simulink model "Hell_ix_Functional_Architecture"  (R2022b)
settings: Solver=VariableStepAuto  StartTime=0.0  StopTime=10.0  RelTol=1e-3
settings Model: Creator=Daniel Sotelo  LastModifiedBy=Daniel Sotelo

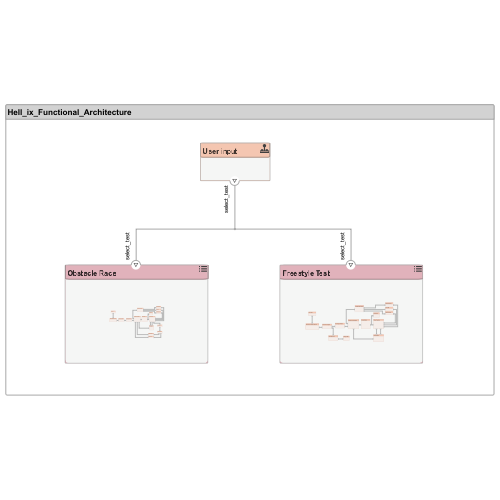
[thumbnail: Simulink's stored preview of the top-level diagram]
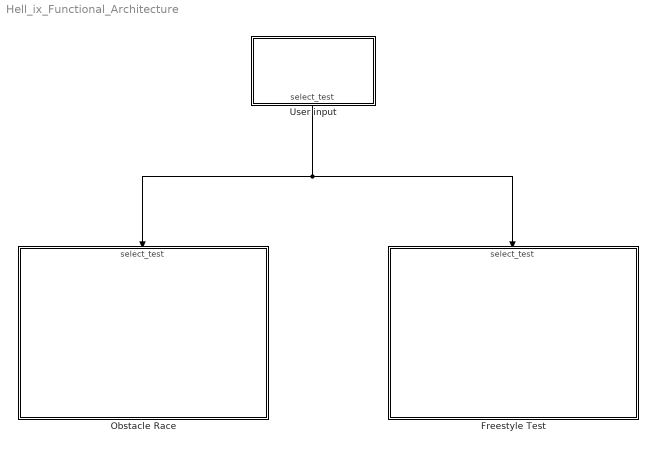
== system Hell_ix_Functional_Architecture ==
  Freestyle Test : Subsystem
      settings: PortSchema="{\"entries\":[{\"content\":{\"headerSize\":26,\"margin\":15,\"minimumSpacing\":25,\"sides\":[{\"content\":{\"connectorIds\":[]},\"type\":\"ConnectorPlacement.EquallySpacedRectSide\",\"uuid\":\"e97e1fd1-9f1b-43cc-bf15-a23fe97b9f57\"},{\"content\":{\"connectorIds\":[],\"side\":\"RIGHT\"},\"type\":\"ConnectorPlacement.EquallySpacedRectSide\",\"uuid\":\"b384b9c5-fcee-4054-b020-18cc4d409726\"},{\"content\":{\"connectorIds\":[\"In1\"],\"side\":\"TOP\"},\"type\":\"ConnectorPlacement.EquallySpacedRectSide\",\"uuid\":\"0ff74274-cc13-4bc9-ab97-befa0144ddb0\"}]},\"type\":\"ConnectorPlacement.EquallySpacedConnector\",\"uuid\":\"32a64cae-dc0e-47e5-be72-f6041fa7e3a1\"}],\"packageUris\":[\"http://schema.mathworks.com/mf0/Connector/R2020b\"],\"version\":\"1.0\"}"
  Obstacle Race : Subsystem
      settings: PortSchema="{\"entries\":[{\"content\":{\"headerSize\":26,\"margin\":15,\"minimumSpacing\":25,\"sides\":[{\"content\":{\"connectorIds\":[]},\"type\":\"ConnectorPlacement.EquallySpacedRectSide\",\"uuid\":\"e97e1fd1-9f1b-43cc-bf15-a23fe97b9f57\"},{\"content\":{\"connectorIds\":[],\"side\":\"RIGHT\"},\"type\":\"ConnectorPlacement.EquallySpacedRectSide\",\"uuid\":\"b384b9c5-fcee-4054-b020-18cc4d409726\"},{\"content\":{\"connectorIds\":[\"In1\"],\"side\":\"TOP\"},\"type\":\"ConnectorPlacement.EquallySpacedRectSide\",\"uuid\":\"0ff74274-cc13-4bc9-ab97-befa0144ddb0\"}]},\"type\":\"ConnectorPlacement.EquallySpacedConnector\",\"uuid\":\"32a64cae-dc0e-47e5-be72-f6041fa7e3a1\"}],\"packageUris\":[\"http://schema.mathworks.com/mf0/Connector/R2020b\"],\"version\":\"1.0\"}"
  User input : Subsystem
      settings: PortSchema="{\"entries\":[{\"content\":{\"headerSize\":26,\"margin\":15,\"minimumSpacing\":25,\"sides\":[{\"content\":{\"connectorIds\":[]},\"type\":\"ConnectorPlacement.EquallySpacedRectSide\",\"uuid\":\"30ce29f3-0e24-4ebf-9153-3e6ba72d02a3\"},{\"content\":{\"connectorIds\":[],\"side\":\"RIGHT\"},\"type\":\"ConnectorPlacement.EquallySpacedRectSide\",\"uuid\":\"fe9b11ce-d1c5-4b81-91f9-8a01d2df3f9c\"},{\"content\":{\"connectorIds\":[],\"side\":\"TOP\"},\"type\":\"ConnectorPlacement.EquallySpacedRectSide\",\"uuid\":\"b1de80d7-4ec1-40a0-acfa-b891e3e0d07e\"},{\"content\":{\"connectorIds\":[\"Out1\"],\"side\":\"BOTTOM\"},\"type\":\"ConnectorPlacement.EquallySpacedRectSide\",\"uuid\":\"e3e43ed0-9352-4cb6-b8e2-474aa3905c46\"}]},\"type\":\"ConnectorPlacement.EquallySpacedConnector\",\"uuid\":\"2db1e156-8200-4f9d-beaf-fd6631afb9bb\"}],\"packageUris\":[\"http://schema.mathworks.com/mf0/Connector/R2020b\"],\"version\":\"1.0\"}"
  wires:
  User input/1(select_test) -> Freestyle Test/1(select_test), Obstacle Race/1(select_test)

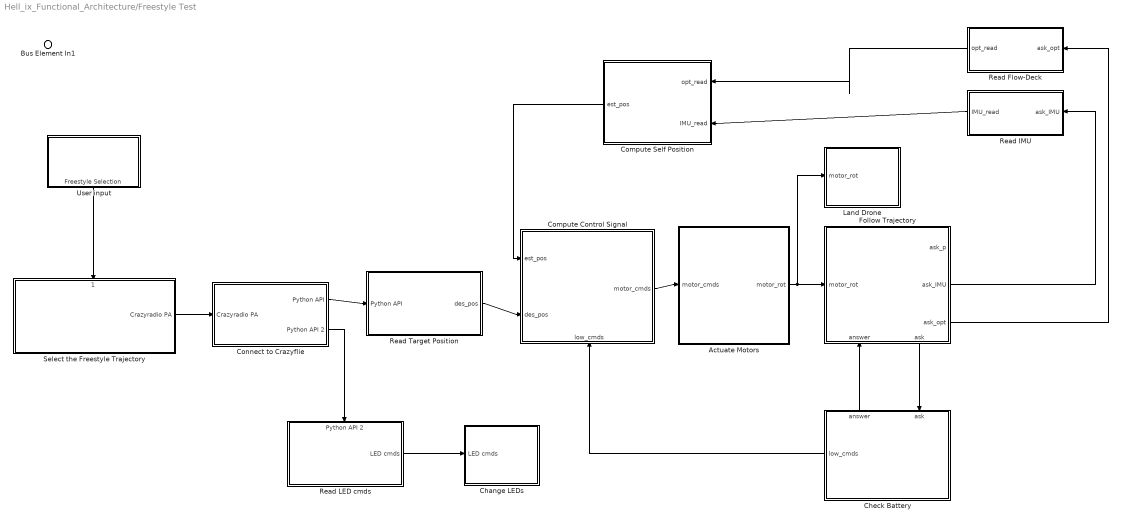
== system Hell_ix_Functional_Architecture/Freestyle Test ==
  Bus Element In1 : Inport  PortName=select_test
  Actuate Motors : Subsystem
      settings: PortSchema="{\"entries\":[{\"content\":{\"headerSize\":26,\"margin\":15,\"minimumSpacing\":25,\"sides\":[{\"content\":{\"connectorIds\":[\"In1\"]},\"type\":\"ConnectorPlacement.EquallySpacedRectSide\",\"uuid\":\"30ce29f3-0e24-4ebf-9153-3e6ba72d02a3\"},{\"content\":{\"connectorIds\":[\"Out1\"],\"side\":\"RIGHT\"},\"type\":\"ConnectorPlacement.EquallySpacedRectSide\",\"uuid\":\"fe9b11ce-d1c5-4b81-91f9-8a01d2df3f9c\"},{\"content\":{\"connectorIds\":[],\"side\":\"TOP\"},\"type\":\"ConnectorPlacement.EquallySpacedRectSide\",\"uuid\":\"b1de80d7-4ec1-40a0-acfa-b891e3e0d07e\"},{\"content\":{\"connectorIds\":[],\"side\":\"BOTTOM\"},\"type\":\"ConnectorPlacement.EquallySpacedRectSide\",\"uuid\":\"15269a5b-ba8a-48cb-be68-3964bc387354\"}]},\"type\":\"ConnectorPlacement.EquallySpacedConnector\",\"uuid\":\"2db1e156-8200-4f9d-beaf-fd6631afb9bb\"}],\"packageUris\":[\"http://schema.mathworks.com/mf0/Connector/R2020b\"],\"version\":\"1.0\"}"
  Change LEDs : Subsystem
      settings: PortSchema="{\"entries\":[{\"content\":{\"headerSize\":26,\"margin\":15,\"minimumSpacing\":25,\"sides\":[{\"content\":{\"connectorIds\":[\"In1\"]},\"type\":\"ConnectorPlacement.EquallySpacedRectSide\",\"uuid\":\"30ce29f3-0e24-4ebf-9153-3e6ba72d02a3\"},{\"content\":{\"connectorIds\":[],\"side\":\"RIGHT\"},\"type\":\"ConnectorPlacement.EquallySpacedRectSide\",\"uuid\":\"fe9b11ce-d1c5-4b81-91f9-8a01d2df3f9c\"},{\"content\":{\"connectorIds\":[],\"side\":\"TOP\"},\"type\":\"ConnectorPlacement.EquallySpacedRectSide\",\"uuid\":\"b1de80d7-4ec1-40a0-acfa-b891e3e0d07e\"}]},\"type\":\"ConnectorPlacement.EquallySpacedConnector\",\"uuid\":\"2db1e156-8200-4f9d-beaf-fd6631afb9bb\"}],\"packageUris\":[\"http://schema.mathworks.com/mf0/Connector/R2020b\"],\"version\":\"1.0\"}"
  Check Battery : Subsystem
      settings: PortSchema="{\"entries\":[{\"content\":{\"headerSize\":26,\"margin\":15,\"minimumSpacing\":25,\"sides\":[{\"content\":{\"connectorIds\":[\"Out1\"]},\"type\":\"ConnectorPlacement.EquallySpacedRectSide\",\"uuid\":\"30ce29f3-0e24-4ebf-9153-3e6ba72d02a3\"},{\"content\":{\"connectorIds\":[],\"side\":\"RIGHT\"},\"type\":\"ConnectorPlacement.EquallySpacedRectSide\",\"uuid\":\"fe9b11ce-d1c5-4b81-91f9-8a01d2df3f9c\"},{\"content\":{\"connectorIds\":[\"Out2\",\"In1\"],\"side\":\"TOP\"},\"type\":\"ConnectorPlacement.EquallySpacedRectSide\",\"uuid\":\"b1de80d7-4ec1-40a0-acfa-b891e3e0d07e\"}]},\"type\":\"ConnectorPlacement.EquallySpacedConnector\",\"uuid\":\"2db1e156-8200-4f9d-beaf-fd6631afb9bb\"}],\"packageUris\":[\"http://schema.mathworks.com/mf0/Connector/R2020b\"],\"version\":\"1.0\"}"
  Compute Control Signal : Subsystem
      settings: PortSchema="{\"entries\":[{\"content\":{\"headerSize\":26,\"margin\":15,\"minimumSpacing\":25,\"sides\":[{\"content\":{\"connectorIds\":[\"In2\",\"In3\"]},\"type\":\"ConnectorPlacement.EquallySpacedRectSide\",\"uuid\":\"30ce29f3-0e24-4ebf-9153-3e6ba72d02a3\"},{\"content\":{\"connectorIds\":[\"Out1\"],\"side\":\"RIGHT\"},\"type\":\"ConnectorPlacement.EquallySpacedRectSide\",\"uuid\":\"fe9b11ce-d1c5-4b81-91f9-8a01d2df3f9c\"},{\"content\":{\"connectorIds\":[],\"side\":\"TOP\"},\"type\":\"ConnectorPlacement.EquallySpacedRectSide\",\"uuid\":\"b1de80d7-4ec1-40a0-acfa-b891e3e0d07e\"},{\"content\":{\"connectorIds\":[\"In1\"],\"side\":\"BOTTOM\"},\"type\":\"ConnectorPlacement.EquallySpacedRectSide\",\"uuid\":\"15269a5b-ba8a-48cb-be68-3964bc387354\"}]},\"type\":\"ConnectorPlacement.EquallySpacedConnector\",\"uuid\":\"2db1e156-8200-4f9d-beaf-fd6631afb9bb\"}],\"packageUris\":[\"http://schema.mathworks.com/mf0/Connector/R2020b\"],\"version\":\"1.0\"}"
  Compute Self Position : Subsystem
      settings: PortSchema="{\"entries\":[{\"content\":{\"headerSize\":26,\"margin\":15,\"minimumSpacing\":25,\"sides\":[{\"content\":{\"connectorIds\":[\"Out1\"]},\"type\":\"ConnectorPlacement.EquallySpacedRectSide\",\"uuid\":\"30ce29f3-0e24-4ebf-9153-3e6ba72d02a3\"},{\"content\":{\"connectorIds\":[\"In1\",\"In2\"],\"side\":\"RIGHT\"},\"type\":\"ConnectorPlacement.EquallySpacedRectSide\",\"uuid\":\"fe9b11ce-d1c5-4b81-91f9-8a01d2df3f9c\"},{\"content\":{\"connectorIds\":[],\"side\":\"TOP\"},\"type\":\"ConnectorPlacement.EquallySpacedRectSide\",\"uuid\":\"b1de80d7-4ec1-40a0-acfa-b891e3e0d07e\"},{\"content\":{\"connectorIds\":[],\"side\":\"BOTTOM\"},\"type\":\"ConnectorPlacement.EquallySpacedRectSide\",\"uuid\":\"463c5264-2d4b-41d6-b420-fe60d6cb1965\"}]},\"type\":\"ConnectorPlacement.EquallySpacedConnector\",\"uuid\":\"2db1e156-8200-4f9d-beaf-fd6631afb9bb\"}],\"packageUris\":[\"http://schema.mathworks.com/mf0/Connector/R2020b\"],\"version\":\"1.0\"}"
  Connect to Crazyflie : Subsystem
      settings: PortSchema="{\"entries\":[{\"content\":{\"headerSize\":26,\"margin\":15,\"minimumSpacing\":25,\"sides\":[{\"content\":{\"connectorIds\":[\"In1\"]},\"type\":\"ConnectorPlacement.EquallySpacedRectSide\",\"uuid\":\"30ce29f3-0e24-4ebf-9153-3e6ba72d02a3\"},{\"content\":{\"connectorIds\":[\"Out1\",\"Out2\"],\"side\":\"RIGHT\"},\"type\":\"ConnectorPlacement.EquallySpacedRectSide\",\"uuid\":\"fe9b11ce-d1c5-4b81-91f9-8a01d2df3f9c\"},{\"content\":{\"connectorIds\":[],\"side\":\"TOP\"},\"type\":\"ConnectorPlacement.EquallySpacedRectSide\",\"uuid\":\"b1de80d7-4ec1-40a0-acfa-b891e3e0d07e\"}]},\"type\":\"ConnectorPlacement.EquallySpacedConnector\",\"uuid\":\"2db1e156-8200-4f9d-beaf-fd6631afb9bb\"}],\"packageUris\":[\"http://schema.mathworks.com/mf0/Connector/R2020b\"],\"version\":\"1.0\"}"
  Follow Trajectory : Subsystem
      settings: PortSchema="{\"entries\":[{\"content\":{\"headerSize\":26,\"margin\":15,\"minimumSpacing\":25,\"sides\":[{\"content\":{\"connectorIds\":[\"In2\"]},\"type\":\"ConnectorPlacement.EquallySpacedRectSide\",\"uuid\":\"30ce29f3-0e24-4ebf-9153-3e6ba72d02a3\"},{\"content\":{\"connectorIds\":[\"Out2\",\"Out1\",\"Out3\"],\"side\":\"RIGHT\"},\"type\":\"ConnectorPlacement.EquallySpacedRectSide\",\"uuid\":\"fe9b11ce-d1c5-4b81-91f9-8a01d2df3f9c\"},{\"content\":{\"connectorIds\":[],\"side\":\"TOP\"},\"type\":\"ConnectorPlacement.EquallySpacedRectSide\",\"uuid\":\"b1de80d7-4ec1-40a0-acfa-b891e3e0d07e\"},{\"content\":{\"connectorIds\":[\"In1\",\"Out4\"],\"side\":\"BOTTOM\"},\"type\":\"ConnectorPlacement.EquallySpacedRectSide\",\"uuid\":\"61505f5d-ae4a-4fe0-ac47-0fc326909193\"}]},\"type\":\"ConnectorPlacement.EquallySpacedConnector\",\"uuid\":\"2db1e156-8200-4f9d-beaf-fd6631afb9bb\"}],\"packageUris\":[\"http://schema.mathworks.com/mf0/Connector/R2020b\"],\"version\":\"1.0\"}"
  Land Drone : Subsystem
      settings: PortSchema="{\"entries\":[{\"content\":{\"headerSize\":26,\"margin\":15,\"minimumSpacing\":25,\"sides\":[{\"content\":{\"connectorIds\":[\"In1\"]},\"type\":\"ConnectorPlacement.EquallySpacedRectSide\",\"uuid\":\"30ce29f3-0e24-4ebf-9153-3e6ba72d02a3\"},{\"content\":{\"connectorIds\":[],\"side\":\"RIGHT\"},\"type\":\"ConnectorPlacement.EquallySpacedRectSide\",\"uuid\":\"fe9b11ce-d1c5-4b81-91f9-8a01d2df3f9c\"},{\"content\":{\"connectorIds\":[],\"side\":\"TOP\"},\"type\":\"ConnectorPlacement.EquallySpacedRectSide\",\"uuid\":\"b1de80d7-4ec1-40a0-acfa-b891e3e0d07e\"}]},\"type\":\"ConnectorPlacement.EquallySpacedConnector\",\"uuid\":\"2db1e156-8200-4f9d-beaf-fd6631afb9bb\"}],\"packageUris\":[\"http://schema.mathworks.com/mf0/Connector/R2020b\"],\"version\":\"1.0\"}"
  Read Flow-Deck : Subsystem
      settings: PortSchema="{\"entries\":[{\"content\":{\"headerSize\":26,\"margin\":15,\"minimumSpacing\":25,\"sides\":[{\"content\":{\"connectorIds\":[\"Out1\"]},\"type\":\"ConnectorPlacement.EquallySpacedRectSide\",\"uuid\":\"30ce29f3-0e24-4ebf-9153-3e6ba72d02a3\"},{\"content\":{\"connectorIds\":[\"In1\"],\"side\":\"RIGHT\"},\"type\":\"ConnectorPlacement.EquallySpacedRectSide\",\"uuid\":\"fe9b11ce-d1c5-4b81-91f9-8a01d2df3f9c\"},{\"content\":{\"connectorIds\":[],\"side\":\"TOP\"},\"type\":\"ConnectorPlacement.EquallySpacedRectSide\",\"uuid\":\"b1de80d7-4ec1-40a0-acfa-b891e3e0d07e\"},{\"content\":{\"connectorIds\":[],\"side\":\"BOTTOM\"},\"type\":\"ConnectorPlacement.EquallySpacedRectSide\",\"uuid\":\"15269a5b-ba8a-48cb-be68-3964bc387354\"}]},\"type\":\"ConnectorPlacement.EquallySpacedConnector\",\"uuid\":\"2db1e156-8200-4f9d-beaf-fd6631afb9bb\"}],\"packageUris\":[\"http://schema.mathworks.com/mf0/Connector/R2020b\"],\"version\":\"1.0\"}"
  Read IMU : Subsystem
      settings: PortSchema="{\"entries\":[{\"content\":{\"headerSize\":26,\"margin\":15,\"minimumSpacing\":25,\"sides\":[{\"content\":{\"connectorIds\":[\"Out1\"]},\"type\":\"ConnectorPlacement.EquallySpacedRectSide\",\"uuid\":\"30ce29f3-0e24-4ebf-9153-3e6ba72d02a3\"},{\"content\":{\"connectorIds\":[\"In1\"],\"side\":\"RIGHT\"},\"type\":\"ConnectorPlacement.EquallySpacedRectSide\",\"uuid\":\"fe9b11ce-d1c5-4b81-91f9-8a01d2df3f9c\"},{\"content\":{\"connectorIds\":[],\"side\":\"TOP\"},\"type\":\"ConnectorPlacement.EquallySpacedRectSide\",\"uuid\":\"b1de80d7-4ec1-40a0-acfa-b891e3e0d07e\"},{\"content\":{\"connectorIds\":[],\"side\":\"BOTTOM\"},\"type\":\"ConnectorPlacement.EquallySpacedRectSide\",\"uuid\":\"15269a5b-ba8a-48cb-be68-3964bc387354\"}]},\"type\":\"ConnectorPlacement.EquallySpacedConnector\",\"uuid\":\"2db1e156-8200-4f9d-beaf-fd6631afb9bb\"}],\"packageUris\":[\"http://schema.mathworks.com/mf0/Connector/R2020b\"],\"version\":\"1.0\"}"
  Read LED cmds : Subsystem
      settings: PortSchema="{\"entries\":[{\"content\":{\"headerSize\":26,\"margin\":15,\"minimumSpacing\":25,\"sides\":[{\"content\":{\"connectorIds\":[]},\"type\":\"ConnectorPlacement.EquallySpacedRectSide\",\"uuid\":\"30ce29f3-0e24-4ebf-9153-3e6ba72d02a3\"},{\"content\":{\"connectorIds\":[\"Out1\"],\"side\":\"RIGHT\"},\"type\":\"ConnectorPlacement.EquallySpacedRectSide\",\"uuid\":\"fe9b11ce-d1c5-4b81-91f9-8a01d2df3f9c\"},{\"content\":{\"connectorIds\":[\"In1\"],\"side\":\"TOP\"},\"type\":\"ConnectorPlacement.EquallySpacedRectSide\",\"uuid\":\"b1de80d7-4ec1-40a0-acfa-b891e3e0d07e\"}]},\"type\":\"ConnectorPlacement.EquallySpacedConnector\",\"uuid\":\"2db1e156-8200-4f9d-beaf-fd6631afb9bb\"}],\"packageUris\":[\"http://schema.mathworks.com/mf0/Connector/R2020b\"],\"version\":\"1.0\"}"
  Read Target Position : Subsystem
      settings: PortSchema="{\"entries\":[{\"content\":{\"headerSize\":26,\"margin\":15,\"minimumSpacing\":25,\"sides\":[{\"content\":{\"connectorIds\":[\"In1\"]},\"type\":\"ConnectorPlacement.EquallySpacedRectSide\",\"uuid\":\"30ce29f3-0e24-4ebf-9153-3e6ba72d02a3\"},{\"content\":{\"connectorIds\":[\"Out1\"],\"side\":\"RIGHT\"},\"type\":\"ConnectorPlacement.EquallySpacedRectSide\",\"uuid\":\"fe9b11ce-d1c5-4b81-91f9-8a01d2df3f9c\"},{\"content\":{\"connectorIds\":[],\"side\":\"TOP\"},\"type\":\"ConnectorPlacement.EquallySpacedRectSide\",\"uuid\":\"b1de80d7-4ec1-40a0-acfa-b891e3e0d07e\"}]},\"type\":\"ConnectorPlacement.EquallySpacedConnector\",\"uuid\":\"2db1e156-8200-4f9d-beaf-fd6631afb9bb\"}],\"packageUris\":[\"http://schema.mathworks.com/mf0/Connector/R2020b\"],\"version\":\"1.0\"}"
  Select the Freestyle Trajectory : Subsystem
      settings: PortSchema="{\"entries\":[{\"content\":{\"headerSize\":26,\"margin\":15,\"minimumSpacing\":25,\"sides\":[{\"content\":{\"connectorIds\":[]},\"type\":\"ConnectorPlacement.EquallySpacedRectSide\",\"uuid\":\"30ce29f3-0e24-4ebf-9153-3e6ba72d02a3\"},{\"content\":{\"connectorIds\":[\"Out1\"],\"side\":\"RIGHT\"},\"type\":\"ConnectorPlacement.EquallySpacedRectSide\",\"uuid\":\"fe9b11ce-d1c5-4b81-91f9-8a01d2df3f9c\"},{\"content\":{\"connectorIds\":[\"In1\"],\"side\":\"TOP\"},\"type\":\"ConnectorPlacement.EquallySpacedRectSide\",\"uuid\":\"b1de80d7-4ec1-40a0-acfa-b891e3e0d07e\"}]},\"type\":\"ConnectorPlacement.EquallySpacedConnector\",\"uuid\":\"2db1e156-8200-4f9d-beaf-fd6631afb9bb\"}],\"packageUris\":[\"http://schema.mathworks.com/mf0/Connector/R2020b\"],\"version\":\"1.0\"}"
  User input : Subsystem
      settings: PortSchema="{\"entries\":[{\"content\":{\"headerSize\":26,\"margin\":15,\"minimumSpacing\":25,\"sides\":[{\"content\":{\"connectorIds\":[]},\"type\":\"ConnectorPlacement.EquallySpacedRectSide\",\"uuid\":\"30ce29f3-0e24-4ebf-9153-3e6ba72d02a3\"},{\"content\":{\"connectorIds\":[],\"side\":\"RIGHT\"},\"type\":\"ConnectorPlacement.EquallySpacedRectSide\",\"uuid\":\"fe9b11ce-d1c5-4b81-91f9-8a01d2df3f9c\"},{\"content\":{\"connectorIds\":[],\"side\":\"TOP\"},\"type\":\"ConnectorPlacement.EquallySpacedRectSide\",\"uuid\":\"b1de80d7-4ec1-40a0-acfa-b891e3e0d07e\"},{\"content\":{\"connectorIds\":[\"Out1\"],\"side\":\"BOTTOM\"},\"type\":\"ConnectorPlacement.EquallySpacedRectSide\",\"uuid\":\"e3e43ed0-9352-4cb6-b8e2-474aa3905c46\"}]},\"type\":\"ConnectorPlacement.EquallySpacedConnector\",\"uuid\":\"2db1e156-8200-4f9d-beaf-fd6631afb9bb\"}],\"packageUris\":[\"http://schema.mathworks.com/mf0/Connector/R2020b\"],\"version\":\"1.0\"}"
  wires:
  Connect to Crazyflie/1(Python API) -> Read Target Position/1(Python API)
  Follow Trajectory/3(ask_opt) -> Read Flow-Deck/1(ask_opt)
  Follow Trajectory/4(ask) -> Check Battery/1(ask)
  User input/1(Freestyle Selection) -> Select the Freestyle Trajectory/1(" ")
  Read Flow-Deck/1(opt_read) -> Compute Self Position/1(opt_read)
  Read Target Position/1(des_pos) -> Compute Control Signal/3(des_pos)
  Check Battery/1(low_cmds) -> Compute Control Signal/1(low_cmds)
  Actuate Motors/1(motor_rot) -> Land Drone/1(motor_rot), Follow Trajectory/2(motor_rot)
  Check Battery/2(answer) -> Follow Trajectory/1(answer)
  Follow Trajectory/1(ask_IMU) -> Read IMU/1(ask_IMU)
  Compute Control Signal/1(motor_cmds) -> Actuate Motors/1(motor_cmds)
  Read IMU/1(IMU_read) -> Compute Self Position/2(IMU_read)
  Select the Freestyle Trajectory/1(Crazyradio PA) -> Connect to Crazyflie/1(Crazyradio PA)
  Compute Self Position/1(est_pos) -> Compute Control Signal/2(est_pos)
  Connect to Crazyflie/2(Python API 2) -> Read LED cmds/1(Python API 2)
  Read LED cmds/1(LED cmds) -> Change LEDs/1(LED cmds)

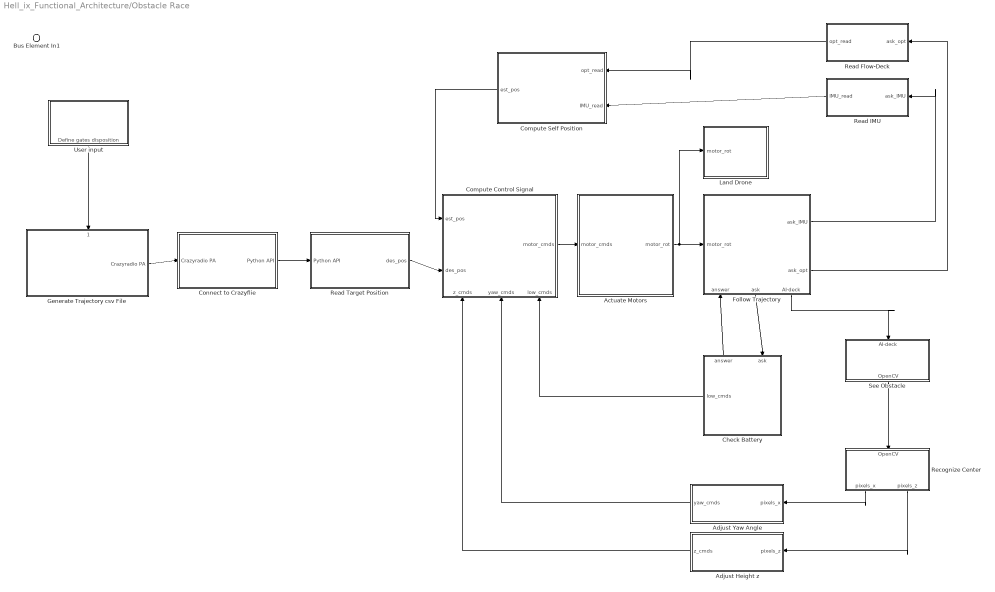
== system Hell_ix_Functional_Architecture/Obstacle Race ==
  Bus Element In1 : Inport  PortName=select_test
  Actuate Motors : Subsystem
      settings: PortSchema="{\"entries\":[{\"content\":{\"headerSize\":26,\"margin\":15,\"minimumSpacing\":25,\"sides\":[{\"content\":{\"connectorIds\":[\"In1\"]},\"type\":\"ConnectorPlacement.EquallySpacedRectSide\",\"uuid\":\"30ce29f3-0e24-4ebf-9153-3e6ba72d02a3\"},{\"content\":{\"connectorIds\":[\"Out1\"],\"side\":\"RIGHT\"},\"type\":\"ConnectorPlacement.EquallySpacedRectSide\",\"uuid\":\"fe9b11ce-d1c5-4b81-91f9-8a01d2df3f9c\"},{\"content\":{\"connectorIds\":[],\"side\":\"TOP\"},\"type\":\"ConnectorPlacement.EquallySpacedRectSide\",\"uuid\":\"b1de80d7-4ec1-40a0-acfa-b891e3e0d07e\"},{\"content\":{\"connectorIds\":[],\"side\":\"BOTTOM\"},\"type\":\"ConnectorPlacement.EquallySpacedRectSide\",\"uuid\":\"15269a5b-ba8a-48cb-be68-3964bc387354\"}]},\"type\":\"ConnectorPlacement.EquallySpacedConnector\",\"uuid\":\"2db1e156-8200-4f9d-beaf-fd6631afb9bb\"}],\"packageUris\":[\"http://schema.mathworks.com/mf0/Connector/R2020b\"],\"version\":\"1.0\"}"
  Adjust Height z : Subsystem
      settings: PortSchema="{\"entries\":[{\"content\":{\"headerSize\":26,\"margin\":15,\"minimumSpacing\":25,\"sides\":[{\"content\":{\"connectorIds\":[\"Out1\"]},\"type\":\"ConnectorPlacement.EquallySpacedRectSide\",\"uuid\":\"30ce29f3-0e24-4ebf-9153-3e6ba72d02a3\"},{\"content\":{\"connectorIds\":[\"In1\"],\"side\":\"RIGHT\"},\"type\":\"ConnectorPlacement.EquallySpacedRectSide\",\"uuid\":\"fe9b11ce-d1c5-4b81-91f9-8a01d2df3f9c\"},{\"content\":{\"connectorIds\":[],\"side\":\"TOP\"},\"type\":\"ConnectorPlacement.EquallySpacedRectSide\",\"uuid\":\"b1de80d7-4ec1-40a0-acfa-b891e3e0d07e\"}]},\"type\":\"ConnectorPlacement.EquallySpacedConnector\",\"uuid\":\"2db1e156-8200-4f9d-beaf-fd6631afb9bb\"}],\"packageUris\":[\"http://schema.mathworks.com/mf0/Connector/R2020b\"],\"version\":\"1.0\"}"
  Adjust Yaw Angle : Subsystem
      settings: PortSchema="{\"entries\":[{\"content\":{\"headerSize\":26,\"margin\":15,\"minimumSpacing\":25,\"sides\":[{\"content\":{\"connectorIds\":[\"Out1\"]},\"type\":\"ConnectorPlacement.EquallySpacedRectSide\",\"uuid\":\"30ce29f3-0e24-4ebf-9153-3e6ba72d02a3\"},{\"content\":{\"connectorIds\":[\"In1\"],\"side\":\"RIGHT\"},\"type\":\"ConnectorPlacement.EquallySpacedRectSide\",\"uuid\":\"fe9b11ce-d1c5-4b81-91f9-8a01d2df3f9c\"},{\"content\":{\"connectorIds\":[],\"side\":\"TOP\"},\"type\":\"ConnectorPlacement.EquallySpacedRectSide\",\"uuid\":\"b1de80d7-4ec1-40a0-acfa-b891e3e0d07e\"}]},\"type\":\"ConnectorPlacement.EquallySpacedConnector\",\"uuid\":\"2db1e156-8200-4f9d-beaf-fd6631afb9bb\"}],\"packageUris\":[\"http://schema.mathworks.com/mf0/Connector/R2020b\"],\"version\":\"1.0\"}"
  Check Battery : Subsystem
      settings: PortSchema="{\"entries\":[{\"content\":{\"headerSize\":26,\"margin\":15,\"minimumSpacing\":25,\"sides\":[{\"content\":{\"connectorIds\":[\"Out1\"]},\"type\":\"ConnectorPlacement.EquallySpacedRectSide\",\"uuid\":\"30ce29f3-0e24-4ebf-9153-3e6ba72d02a3\"},{\"content\":{\"connectorIds\":[],\"side\":\"RIGHT\"},\"type\":\"ConnectorPlacement.EquallySpacedRectSide\",\"uuid\":\"fe9b11ce-d1c5-4b81-91f9-8a01d2df3f9c\"},{\"content\":{\"connectorIds\":[\"Out2\",\"In1\"],\"side\":\"TOP\"},\"type\":\"ConnectorPlacement.EquallySpacedRectSide\",\"uuid\":\"b1de80d7-4ec1-40a0-acfa-b891e3e0d07e\"}]},\"type\":\"ConnectorPlacement.EquallySpacedConnector\",\"uuid\":\"2db1e156-8200-4f9d-beaf-fd6631afb9bb\"}],\"packageUris\":[\"http://schema.mathworks.com/mf0/Connector/R2020b\"],\"version\":\"1.0\"}"
  Compute Control Signal : Subsystem
      settings: PortSchema="{\"entries\":[{\"content\":{\"headerSize\":26,\"margin\":15,\"minimumSpacing\":25,\"sides\":[{\"content\":{\"connectorIds\":[\"In4\",\"In5\"]},\"type\":\"ConnectorPlacement.EquallySpacedRectSide\",\"uuid\":\"30ce29f3-0e24-4ebf-9153-3e6ba72d02a3\"},{\"content\":{\"connectorIds\":[\"Out1\"],\"side\":\"RIGHT\"},\"type\":\"ConnectorPlacement.EquallySpacedRectSide\",\"uuid\":\"fe9b11ce-d1c5-4b81-91f9-8a01d2df3f9c\"},{\"content\":{\"connectorIds\":[],\"side\":\"TOP\"},\"type\":\"ConnectorPlacement.EquallySpacedRectSide\",\"uuid\":\"b1de80d7-4ec1-40a0-acfa-b891e3e0d07e\"},{\"content\":{\"connectorIds\":[\"In1\",\"In2\",\"In3\"],\"side\":\"BOTTOM\"},\"type\":\"ConnectorPlacement.EquallySpacedRectSide\",\"uuid\":\"15269a5b-ba8a-48cb-be68-3964bc387354\"}]},\"type\":\"ConnectorPlacement.EquallySpacedConnector\",\"uuid\":\"2db1e156-8200-4f9d-beaf-fd6631afb9bb\"}],\"packageUris\":[\"http://schema.mathworks.com/mf0/Connector/R2020b\"],\"version\":\"1.0\"}"
  Compute Self Position : Subsystem
      settings: PortSchema="{\"entries\":[{\"content\":{\"headerSize\":26,\"margin\":15,\"minimumSpacing\":25,\"sides\":[{\"content\":{\"connectorIds\":[\"Out1\"]},\"type\":\"ConnectorPlacement.EquallySpacedRectSide\",\"uuid\":\"30ce29f3-0e24-4ebf-9153-3e6ba72d02a3\"},{\"content\":{\"connectorIds\":[\"In1\",\"In2\"],\"side\":\"RIGHT\"},\"type\":\"ConnectorPlacement.EquallySpacedRectSide\",\"uuid\":\"fe9b11ce-d1c5-4b81-91f9-8a01d2df3f9c\"},{\"content\":{\"connectorIds\":[],\"side\":\"TOP\"},\"type\":\"ConnectorPlacement.EquallySpacedRectSide\",\"uuid\":\"b1de80d7-4ec1-40a0-acfa-b891e3e0d07e\"},{\"content\":{\"connectorIds\":[],\"side\":\"BOTTOM\"},\"type\":\"ConnectorPlacement.EquallySpacedRectSide\",\"uuid\":\"463c5264-2d4b-41d6-b420-fe60d6cb1965\"}]},\"type\":\"ConnectorPlacement.EquallySpacedConnector\",\"uuid\":\"2db1e156-8200-4f9d-beaf-fd6631afb9bb\"}],\"packageUris\":[\"http://schema.mathworks.com/mf0/Connector/R2020b\"],\"version\":\"1.0\"}"
  Connect to Crazyflie : Subsystem
      settings: PortSchema="{\"entries\":[{\"content\":{\"headerSize\":26,\"margin\":15,\"minimumSpacing\":25,\"sides\":[{\"content\":{\"connectorIds\":[\"In1\"]},\"type\":\"ConnectorPlacement.EquallySpacedRectSide\",\"uuid\":\"30ce29f3-0e24-4ebf-9153-3e6ba72d02a3\"},{\"content\":{\"connectorIds\":[\"Out1\"],\"side\":\"RIGHT\"},\"type\":\"ConnectorPlacement.EquallySpacedRectSide\",\"uuid\":\"fe9b11ce-d1c5-4b81-91f9-8a01d2df3f9c\"},{\"content\":{\"connectorIds\":[],\"side\":\"TOP\"},\"type\":\"ConnectorPlacement.EquallySpacedRectSide\",\"uuid\":\"b1de80d7-4ec1-40a0-acfa-b891e3e0d07e\"}]},\"type\":\"ConnectorPlacement.EquallySpacedConnector\",\"uuid\":\"2db1e156-8200-4f9d-beaf-fd6631afb9bb\"}],\"packageUris\":[\"http://schema.mathworks.com/mf0/Connector/R2020b\"],\"version\":\"1.0\"}"
  Follow Trajectory : Subsystem
      settings: PortSchema="{\"entries\":[{\"content\":{\"headerSize\":26,\"margin\":15,\"minimumSpacing\":25,\"sides\":[{\"content\":{\"connectorIds\":[\"In2\"]},\"type\":\"ConnectorPlacement.EquallySpacedRectSide\",\"uuid\":\"30ce29f3-0e24-4ebf-9153-3e6ba72d02a3\"},{\"content\":{\"connectorIds\":[\"Out2\",\"Out3\"],\"side\":\"RIGHT\"},\"type\":\"ConnectorPlacement.EquallySpacedRectSide\",\"uuid\":\"fe9b11ce-d1c5-4b81-91f9-8a01d2df3f9c\"},{\"content\":{\"connectorIds\":[],\"side\":\"TOP\"},\"type\":\"ConnectorPlacement.EquallySpacedRectSide\",\"uuid\":\"b1de80d7-4ec1-40a0-acfa-b891e3e0d07e\"},{\"content\":{\"connectorIds\":[\"In1\",\"Out4\",\"Out1\"],\"side\":\"BOTTOM\"},\"type\":\"ConnectorPlacement.EquallySpacedRectSide\",\"uuid\":\"61505f5d-ae4a-4fe0-ac47-0fc326909193\"}]},\"type\":\"ConnectorPlacement.EquallySpacedConnector\",\"uuid\":\"2db1e156-8200-4f9d-beaf-fd6631afb9bb\"}],\"packageUris\":[\"http://schema.mathworks.com/mf0/Connector/R2020b\"],\"version\":\"1.0\"}"
  Generate Trajectory csv File : Subsystem
      settings: PortSchema="{\"entries\":[{\"content\":{\"headerSize\":26,\"margin\":15,\"minimumSpacing\":25,\"sides\":[{\"content\":{\"connectorIds\":[]},\"type\":\"ConnectorPlacement.EquallySpacedRectSide\",\"uuid\":\"30ce29f3-0e24-4ebf-9153-3e6ba72d02a3\"},{\"content\":{\"connectorIds\":[\"Out1\"],\"side\":\"RIGHT\"},\"type\":\"ConnectorPlacement.EquallySpacedRectSide\",\"uuid\":\"fe9b11ce-d1c5-4b81-91f9-8a01d2df3f9c\"},{\"content\":{\"connectorIds\":[\"In1\"],\"side\":\"TOP\"},\"type\":\"ConnectorPlacement.EquallySpacedRectSide\",\"uuid\":\"b1de80d7-4ec1-40a0-acfa-b891e3e0d07e\"}]},\"type\":\"ConnectorPlacement.EquallySpacedConnector\",\"uuid\":\"2db1e156-8200-4f9d-beaf-fd6631afb9bb\"}],\"packageUris\":[\"http://schema.mathworks.com/mf0/Connector/R2020b\"],\"version\":\"1.0\"}"
  Land Drone : Subsystem
      settings: PortSchema="{\"entries\":[{\"content\":{\"headerSize\":26,\"margin\":15,\"minimumSpacing\":25,\"sides\":[{\"content\":{\"connectorIds\":[\"In1\"]},\"type\":\"ConnectorPlacement.EquallySpacedRectSide\",\"uuid\":\"30ce29f3-0e24-4ebf-9153-3e6ba72d02a3\"},{\"content\":{\"connectorIds\":[],\"side\":\"RIGHT\"},\"type\":\"ConnectorPlacement.EquallySpacedRectSide\",\"uuid\":\"fe9b11ce-d1c5-4b81-91f9-8a01d2df3f9c\"},{\"content\":{\"connectorIds\":[],\"side\":\"TOP\"},\"type\":\"ConnectorPlacement.EquallySpacedRectSide\",\"uuid\":\"b1de80d7-4ec1-40a0-acfa-b891e3e0d07e\"}]},\"type\":\"ConnectorPlacement.EquallySpacedConnector\",\"uuid\":\"2db1e156-8200-4f9d-beaf-fd6631afb9bb\"}],\"packageUris\":[\"http://schema.mathworks.com/mf0/Connector/R2020b\"],\"version\":\"1.0\"}"
  Read Flow-Deck : Subsystem
      settings: PortSchema="{\"entries\":[{\"content\":{\"headerSize\":26,\"margin\":15,\"minimumSpacing\":25,\"sides\":[{\"content\":{\"connectorIds\":[\"Out1\"]},\"type\":\"ConnectorPlacement.EquallySpacedRectSide\",\"uuid\":\"30ce29f3-0e24-4ebf-9153-3e6ba72d02a3\"},{\"content\":{\"connectorIds\":[\"In1\"],\"side\":\"RIGHT\"},\"type\":\"ConnectorPlacement.EquallySpacedRectSide\",\"uuid\":\"fe9b11ce-d1c5-4b81-91f9-8a01d2df3f9c\"},{\"content\":{\"connectorIds\":[],\"side\":\"TOP\"},\"type\":\"ConnectorPlacement.EquallySpacedRectSide\",\"uuid\":\"b1de80d7-4ec1-40a0-acfa-b891e3e0d07e\"},{\"content\":{\"connectorIds\":[],\"side\":\"BOTTOM\"},\"type\":\"ConnectorPlacement.EquallySpacedRectSide\",\"uuid\":\"15269a5b-ba8a-48cb-be68-3964bc387354\"}]},\"type\":\"ConnectorPlacement.EquallySpacedConnector\",\"uuid\":\"2db1e156-8200-4f9d-beaf-fd6631afb9bb\"}],\"packageUris\":[\"http://schema.mathworks.com/mf0/Connector/R2020b\"],\"version\":\"1.0\"}"
  Read IMU : Subsystem
      settings: PortSchema="{\"entries\":[{\"content\":{\"headerSize\":26,\"margin\":15,\"minimumSpacing\":25,\"sides\":[{\"content\":{\"connectorIds\":[\"Out1\"]},\"type\":\"ConnectorPlacement.EquallySpacedRectSide\",\"uuid\":\"30ce29f3-0e24-4ebf-9153-3e6ba72d02a3\"},{\"content\":{\"connectorIds\":[\"In1\"],\"side\":\"RIGHT\"},\"type\":\"ConnectorPlacement.EquallySpacedRectSide\",\"uuid\":\"fe9b11ce-d1c5-4b81-91f9-8a01d2df3f9c\"},{\"content\":{\"connectorIds\":[],\"side\":\"TOP\"},\"type\":\"ConnectorPlacement.EquallySpacedRectSide\",\"uuid\":\"b1de80d7-4ec1-40a0-acfa-b891e3e0d07e\"},{\"content\":{\"connectorIds\":[],\"side\":\"BOTTOM\"},\"type\":\"ConnectorPlacement.EquallySpacedRectSide\",\"uuid\":\"15269a5b-ba8a-48cb-be68-3964bc387354\"}]},\"type\":\"ConnectorPlacement.EquallySpacedConnector\",\"uuid\":\"2db1e156-8200-4f9d-beaf-fd6631afb9bb\"}],\"packageUris\":[\"http://schema.mathworks.com/mf0/Connector/R2020b\"],\"version\":\"1.0\"}"
  Read Target Position : Subsystem
      settings: PortSchema="{\"entries\":[{\"content\":{\"headerSize\":26,\"margin\":15,\"minimumSpacing\":25,\"sides\":[{\"content\":{\"connectorIds\":[\"In1\"]},\"type\":\"ConnectorPlacement.EquallySpacedRectSide\",\"uuid\":\"30ce29f3-0e24-4ebf-9153-3e6ba72d02a3\"},{\"content\":{\"connectorIds\":[\"Out1\"],\"side\":\"RIGHT\"},\"type\":\"ConnectorPlacement.EquallySpacedRectSide\",\"uuid\":\"fe9b11ce-d1c5-4b81-91f9-8a01d2df3f9c\"},{\"content\":{\"connectorIds\":[],\"side\":\"TOP\"},\"type\":\"ConnectorPlacement.EquallySpacedRectSide\",\"uuid\":\"b1de80d7-4ec1-40a0-acfa-b891e3e0d07e\"}]},\"type\":\"ConnectorPlacement.EquallySpacedConnector\",\"uuid\":\"2db1e156-8200-4f9d-beaf-fd6631afb9bb\"}],\"packageUris\":[\"http://schema.mathworks.com/mf0/Connector/R2020b\"],\"version\":\"1.0\"}"
  Recognize Center : Subsystem
      settings: PortSchema="{\"entries\":[{\"content\":{\"headerSize\":26,\"margin\":15,\"minimumSpacing\":25,\"sides\":[{\"content\":{\"connectorIds\":[]},\"type\":\"ConnectorPlacement.EquallySpacedRectSide\",\"uuid\":\"30ce29f3-0e24-4ebf-9153-3e6ba72d02a3\"},{\"content\":{\"connectorIds\":[],\"side\":\"RIGHT\"},\"type\":\"ConnectorPlacement.EquallySpacedRectSide\",\"uuid\":\"fe9b11ce-d1c5-4b81-91f9-8a01d2df3f9c\"},{\"content\":{\"connectorIds\":[\"In1\"],\"side\":\"TOP\"},\"type\":\"ConnectorPlacement.EquallySpacedRectSide\",\"uuid\":\"b1de80d7-4ec1-40a0-acfa-b891e3e0d07e\"},{\"content\":{\"connectorIds\":[\"Out1\",\"Out2\"],\"side\":\"BOTTOM\"},\"type\":\"ConnectorPlacement.EquallySpacedRectSide\",\"uuid\":\"5e75c728-9af2-4205-b387-daa129fc2d53\"}]},\"type\":\"ConnectorPlacement.EquallySpacedConnector\",\"uuid\":\"2db1e156-8200-4f9d-beaf-fd6631afb9bb\"}],\"packageUris\":[\"http://schema.mathworks.com/mf0/Connector/R2020b\"],\"version\":\"1.0\"}"
  See Obstacle : Subsystem
      settings: PortSchema="{\"entries\":[{\"content\":{\"headerSize\":26,\"margin\":15,\"minimumSpacing\":25,\"sides\":[{\"content\":{\"connectorIds\":[]},\"type\":\"ConnectorPlacement.EquallySpacedRectSide\",\"uuid\":\"30ce29f3-0e24-4ebf-9153-3e6ba72d02a3\"},{\"content\":{\"connectorIds\":[],\"side\":\"RIGHT\"},\"type\":\"ConnectorPlacement.EquallySpacedRectSide\",\"uuid\":\"fe9b11ce-d1c5-4b81-91f9-8a01d2df3f9c\"},{\"content\":{\"connectorIds\":[\"In1\"],\"side\":\"TOP\"},\"type\":\"ConnectorPlacement.EquallySpacedRectSide\",\"uuid\":\"b1de80d7-4ec1-40a0-acfa-b891e3e0d07e\"},{\"content\":{\"connectorIds\":[\"Out1\"],\"side\":\"BOTTOM\"},\"type\":\"ConnectorPlacement.EquallySpacedRectSide\",\"uuid\":\"12e53c62-2dd7-4016-b718-945882d89040\"}]},\"type\":\"ConnectorPlacement.EquallySpacedConnector\",\"uuid\":\"2db1e156-8200-4f9d-beaf-fd6631afb9bb\"}],\"packageUris\":[\"http://schema.mathworks.com/mf0/Connector/R2020b\"],\"version\":\"1.0\"}"
  User input : Subsystem
      settings: PortSchema="{\"entries\":[{\"content\":{\"headerSize\":26,\"margin\":15,\"minimumSpacing\":25,\"sides\":[{\"content\":{\"connectorIds\":[]},\"type\":\"ConnectorPlacement.EquallySpacedRectSide\",\"uuid\":\"30ce29f3-0e24-4ebf-9153-3e6ba72d02a3\"},{\"content\":{\"connectorIds\":[],\"side\":\"RIGHT\"},\"type\":\"ConnectorPlacement.EquallySpacedRectSide\",\"uuid\":\"fe9b11ce-d1c5-4b81-91f9-8a01d2df3f9c\"},{\"content\":{\"connectorIds\":[],\"side\":\"TOP\"},\"type\":\"ConnectorPlacement.EquallySpacedRectSide\",\"uuid\":\"b1de80d7-4ec1-40a0-acfa-b891e3e0d07e\"},{\"content\":{\"connectorIds\":[\"Out1\"],\"side\":\"BOTTOM\"},\"type\":\"ConnectorPlacement.EquallySpacedRectSide\",\"uuid\":\"e3e43ed0-9352-4cb6-b8e2-474aa3905c46\"}]},\"type\":\"ConnectorPlacement.EquallySpacedConnector\",\"uuid\":\"2db1e156-8200-4f9d-beaf-fd6631afb9bb\"}],\"packageUris\":[\"http://schema.mathworks.com/mf0/Connector/R2020b\"],\"version\":\"1.0\"}"
  wires:
  Connect to Crazyflie/1(Python API) -> Read Target Position/1(Python API)
  Recognize Center/1(pixels_x) -> Adjust Yaw Angle/1(pixels_x)
  Follow Trajectory/3(ask_opt) -> Read Flow-Deck/1(ask_opt)
  Adjust Height z/1(z_cmds) -> Compute Control Signal/1(z_cmds)
  Follow Trajectory/4(ask) -> Check Battery/1(ask)
  User input/1(Define gates disposition) -> Generate Trajectory csv File/1(" ")
  See Obstacle/1(OpenCV) -> Recognize Center/1(OpenCV)
  Recognize Center/2(pixels_z) -> Adjust Height z/1(pixels_z)
  Read Flow-Deck/1(opt_read) -> Compute Self Position/1(opt_read)
  Read Target Position/1(des_pos) -> Compute Control Signal/5(des_pos)
  Check Battery/1(low_cmds) -> Compute Control Signal/3(low_cmds)
  Actuate Motors/1(motor_rot) -> Land Drone/1(motor_rot), Follow Trajectory/2(motor_rot)
  Follow Trajectory/1(AI-deck) -> See Obstacle/1(AI-deck)
  Check Battery/2(answer) -> Follow Trajectory/1(answer)
  Follow Trajectory/2(ask_IMU) -> Read IMU/1(ask_IMU)
  Adjust Yaw Angle/1(yaw_cmds) -> Compute Control Signal/2(yaw_cmds)
  Compute Control Signal/1(motor_cmds) -> Actuate Motors/1(motor_cmds)
  Read IMU/1(IMU_read) -> Compute Self Position/2(IMU_read)
  Generate Trajectory csv File/1(Crazyradio PA) -> Connect to Crazyflie/1(Crazyradio PA)
  Compute Self Position/1(est_pos) -> Compute Control Signal/4(est_pos)

== system Hell_ix_Functional_Architecture/User input ==
  Bus Element Out1 : Outport  PortName=select_test

== system Hell_ix_Functional_Architecture/Freestyle Test/Actuate Motors ==
  Bus Element In1 : Inport  PortName=motor_cmds
  Bus Element Out1 : Outport  PortName=motor_rot

== system Hell_ix_Functional_Architecture/Freestyle Test/Change LEDs ==
  Bus Element In2 : Inport  PortName=LED cmds

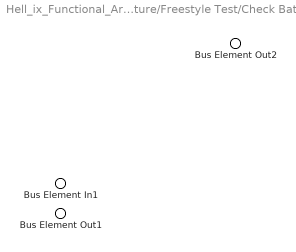
== system Hell_ix_Functional_Architecture/Freestyle Test/Check Battery ==
  Bus Element In1 : Inport  PortName=ask
  Bus Element Out2 : Outport  PortName=low_cmds
  Bus Element Out1 : Outport  Port=2  PortName=answer

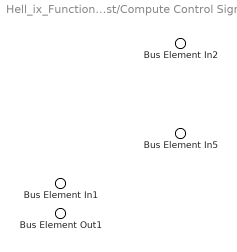
== system Hell_ix_Functional_Architecture/Freestyle Test/Compute Control Signal ==
  Bus Element In5 : Inport  PortName=low_cmds
  Bus Element In2 : Inport  Port=2  PortName=est_pos
  Bus Element In1 : Inport  Port=3  PortName=des_pos
  Bus Element Out1 : Outport  PortName=motor_cmds

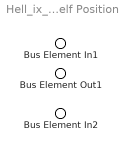
== system Hell_ix_Functional_Architecture/Freestyle Test/Compute Self Position ==
  Bus Element In1 : Inport  PortName=opt_read
  Bus Element In2 : Inport  Port=2  PortName=IMU_read
  Bus Element Out1 : Outport  PortName=est_pos

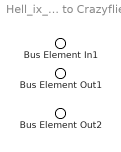
== system Hell_ix_Functional_Architecture/Freestyle Test/Connect to Crazyflie ==
  Bus Element In1 : Inport  PortName=Crazyradio PA
  Bus Element Out1 : Outport  PortName=Python API
  Bus Element Out2 : Outport  Port=2  PortName=Python API 2

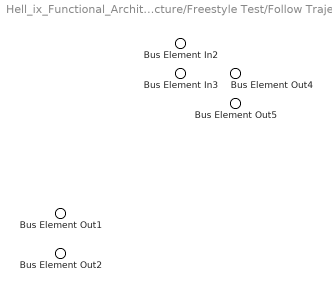
== system Hell_ix_Functional_Architecture/Freestyle Test/Follow Trajectory ==
  Bus Element In3 : Inport  PortName=answer
  Bus Element In2 : Inport  Port=2  PortName=motor_rot
  Bus Element Out4 : Outport  PortName=ask_IMU
  Bus Element Out5 : Outport  Port=2  PortName=ask_p
  Bus Element Out1 : Outport  Port=3  PortName=ask_opt
  Bus Element Out2 : Outport  Port=4  PortName=ask

== system Hell_ix_Functional_Architecture/Freestyle Test/Land Drone ==
  Bus Element In2 : Inport  PortName=motor_rot

== system Hell_ix_Functional_Architecture/Freestyle Test/Read Flow-Deck ==
  Bus Element In1 : Inport  PortName=ask_opt
  Bus Element Out1 : Outport  PortName=opt_read

== system Hell_ix_Functional_Architecture/Freestyle Test/Read IMU ==
  Bus Element In1 : Inport  PortName=ask_IMU
  Bus Element Out1 : Outport  PortName=IMU_read

== system Hell_ix_Functional_Architecture/Freestyle Test/Read LED cmds ==
  Bus Element In1 : Inport  PortName=Python API 2
  Bus Element Out1 : Outport  PortName=LED cmds

== system Hell_ix_Functional_Architecture/Freestyle Test/Read Target Position ==
  Bus Element In1 : Inport  PortName=Python API
  Bus Element Out1 : Outport  PortName=des_pos

== system Hell_ix_Functional_Architecture/Freestyle Test/Select the Freestyle Trajectory ==
  Bus Element In1 : Inport  PortName=""
  Bus Element Out1 : Outport  PortName=Crazyradio PA

== system Hell_ix_Functional_Architecture/Freestyle Test/User input ==
  Bus Element Out1 : Outport  PortName=Freestyle Selection

== system Hell_ix_Functional_Architecture/Obstacle Race/Actuate Motors ==
  Bus Element In1 : Inport  PortName=motor_cmds
  Bus Element Out1 : Outport  PortName=motor_rot

== system Hell_ix_Functional_Architecture/Obstacle Race/Adjust Height z ==
  Bus Element In1 : Inport  PortName=pixels_z
  Bus Element Out1 : Outport  PortName=z_cmds

== system Hell_ix_Functional_Architecture/Obstacle Race/Adjust Yaw Angle ==
  Bus Element In1 : Inport  PortName=pixels_x
  Bus Element Out1 : Outport  PortName=yaw_cmds

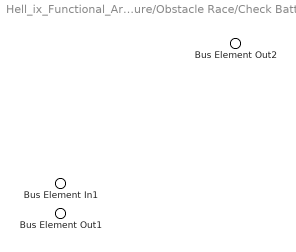
== system Hell_ix_Functional_Architecture/Obstacle Race/Check Battery ==
  Bus Element In1 : Inport  PortName=ask
  Bus Element Out2 : Outport  PortName=low_cmds
  Bus Element Out1 : Outport  Port=2  PortName=answer

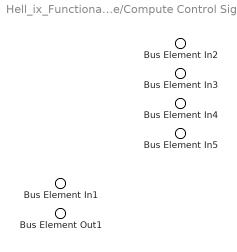
== system Hell_ix_Functional_Architecture/Obstacle Race/Compute Control Signal ==
  Bus Element In4 : Inport  PortName=z_cmds
  Bus Element In3 : Inport  Port=2  PortName=yaw_cmds
  Bus Element In5 : Inport  Port=3  PortName=low_cmds
  Bus Element In2 : Inport  Port=4  PortName=est_pos
  Bus Element In1 : Inport  Port=5  PortName=des_pos
  Bus Element Out1 : Outport  PortName=motor_cmds

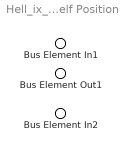
== system Hell_ix_Functional_Architecture/Obstacle Race/Compute Self Position ==
  Bus Element In1 : Inport  PortName=opt_read
  Bus Element In2 : Inport  Port=2  PortName=IMU_read
  Bus Element Out1 : Outport  PortName=est_pos

== system Hell_ix_Functional_Architecture/Obstacle Race/Connect to Crazyflie ==
  Bus Element In1 : Inport  PortName=Crazyradio PA
  Bus Element Out1 : Outport  PortName=Python API

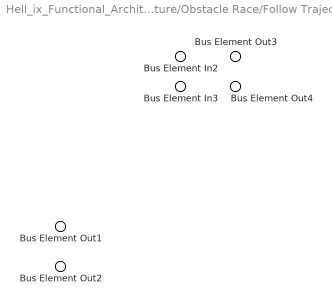
== system Hell_ix_Functional_Architecture/Obstacle Race/Follow Trajectory ==
  Bus Element In3 : Inport  PortName=answer
  Bus Element In2 : Inport  Port=2  PortName=motor_rot
  Bus Element Out3 : Outport  PortName=AI-deck
  Bus Element Out4 : Outport  Port=2  PortName=ask_IMU
  Bus Element Out1 : Outport  Port=3  PortName=ask_opt
  Bus Element Out2 : Outport  Port=4  PortName=ask

== system Hell_ix_Functional_Architecture/Obstacle Race/Generate Trajectory csv File ==
  Bus Element In1 : Inport  PortName=""
  Bus Element Out1 : Outport  PortName=Crazyradio PA

== system Hell_ix_Functional_Architecture/Obstacle Race/Land Drone ==
  Bus Element In2 : Inport  PortName=motor_rot

== system Hell_ix_Functional_Architecture/Obstacle Race/Read Flow-Deck ==
  Bus Element In1 : Inport  PortName=ask_opt
  Bus Element Out1 : Outport  PortName=opt_read

== system Hell_ix_Functional_Architecture/Obstacle Race/Read IMU ==
  Bus Element In1 : Inport  PortName=ask_IMU
  Bus Element Out1 : Outport  PortName=IMU_read

== system Hell_ix_Functional_Architecture/Obstacle Race/Read Target Position ==
  Bus Element In1 : Inport  PortName=Python API
  Bus Element Out1 : Outport  PortName=des_pos

== system Hell_ix_Functional_Architecture/Obstacle Race/Recognize Center ==
  Bus Element In1 : Inport  PortName=OpenCV
  Bus Element Out1 : Outport  PortName=pixels_x
  Bus Element Out2 : Outport  Port=2  PortName=pixels_z

== system Hell_ix_Functional_Architecture/Obstacle Race/See Obstacle ==
  Bus Element In1 : Inport  PortName=AI-deck
  Bus Element Out1 : Outport  PortName=OpenCV

== system Hell_ix_Functional_Architecture/Obstacle Race/User input ==
  Bus Element Out1 : Outport  PortName=Define gates disposition
